simulink model "Pacejka_lateral_tyre_model"  (R2022b)
settings: Solver=VariableStepAuto  StartTime=0.0  StopTime=10.0  RelTol=1e-3
values from neighbouring files (symbols this model uses):
  a1 = -1e-5    (= -1e-05)    [Longitudinal_braking_parameters.m]    (also in Longitudinal_driving_parameters.m; Pacejka_lateral_parameters.m)
  a2 = 1.25    [Longitudinal_braking_parameters.m]    (also in Longitudinal_driving_parameters.m; Pacejka_lateral_parameters.m)
  B = 4.1576    [Longitudinal_braking_parameters.m]    (also in Longitudinal_driving_parameters.m = 5.7507; Pacejka_lateral_parameters.m = 0.1453)
  C = 1.7180    (= 1.718)    [Longitudinal_braking_parameters.m]    (also in Longitudinal_driving_parameters.m = 1.2421; Pacejka_lateral_parameters.m = 1.5511)
settings Model: Creator=webstert  LastModifiedBy=webstert

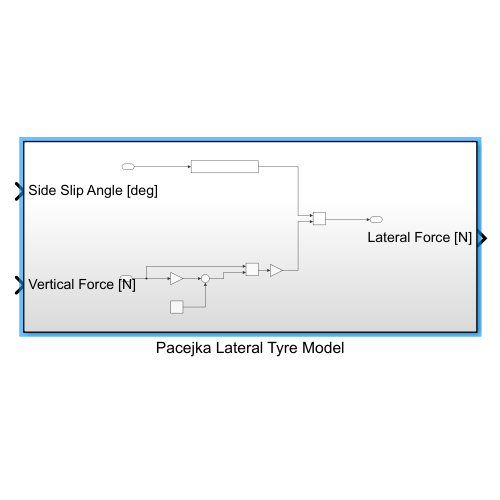
[thumbnail: Simulink's stored preview of the top-level diagram]
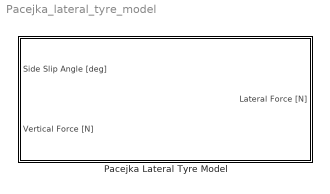
== system Pacejka_lateral_tyre_model ==
  Pacejka Lateral Tyre Model : Subsystem

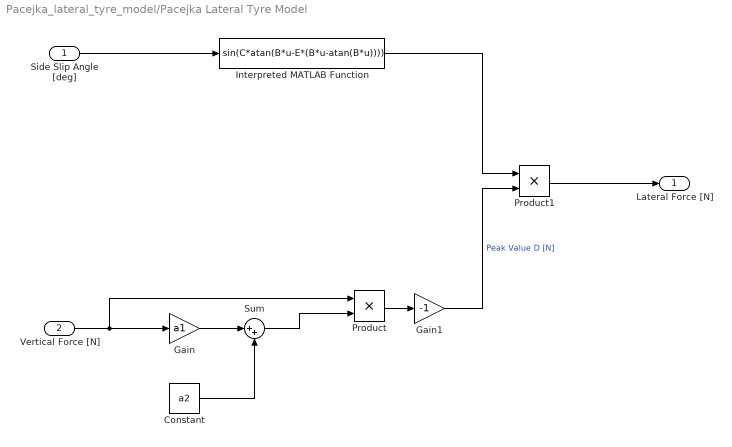
== system Pacejka_lateral_tyre_model/Pacejka Lateral Tyre Model ==
  Side Slip Angle [deg] : Inport
  Vertical Force [N] : Inport  Port=2
  Constant : Constant  Value=a2
  Gain : Gain  Gain=a1
  Gain1 : Gain  Gain=-1
  Interpreted MATLAB Function : MATLABFcn  MATLABFcn=sin(C*atan(B*u-E*(B*u-atan(B*u))))
  Product : Product
  Product1 : Product
  Sum : Sum  Inputs=|++
  Lateral Force [N] : Outport
  wires:
  Vertical Force [N]/1 -> Product/1, Gain/1
  Constant/1 -> Sum/2
  Gain/1 -> Sum/1
  Sum/1 -> Product/2
  Product/1 -> Gain1/1
  Gain1/1 -> Product1/2  "Peak Value D [N]"
  Side Slip Angle [deg]/1 -> Interpreted MATLAB Function/1
  Interpreted MATLAB Function/1 -> Product1/1
  Product1/1 -> Lateral Force [N]/1
